simulink model "a"  (R2022a)
settings: Solver=VariableStepAuto  StartTime=0.0  StopTime=0.1  RelTol=1e-3
libraries: commrandsrc3 x1, dspsrcs4 x1
(part 4 of 4)

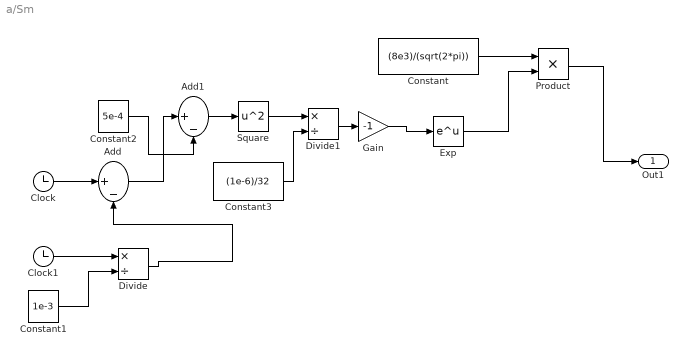
== system a/Sm ==
  Add : Sum  Inputs=|+-
  Add1 : Sum  Inputs=|+-
  Clock : Clock
  Clock1 : Clock
  Constant : Constant  Value=(8e3)/(sqrt(2*pi))
  Constant1 : Constant  Value=1e-3
  Constant2 : Constant  Value=5e-4
  Constant3 : Constant  Value=(1e-6)/32
  Divide : Product  Inputs=*/
  Divide1 : Product  Inputs=*/
  Exp : Math
  Gain : Gain  Gain=-1
  Product : Product
  Square : Math  Operator=square
  Out1 : Outport
  wires:
  Constant/1 -> Product/1
  Exp/1 -> Product/2
  Clock/1 -> Add/1
  Clock1/1 -> Divide/1
  Constant1/1 -> Divide/2
  Divide/1 -> Add/2
  Constant2/1 -> Add1/2
  Add/1 -> Add1/1
  Add1/1 -> Square/1
  Square/1 -> Divide1/1
  Constant3/1 -> Divide1/2
  Divide1/1 -> Gain/1
  Gain/1 -> Exp/1
  Product/1 -> Out1/1

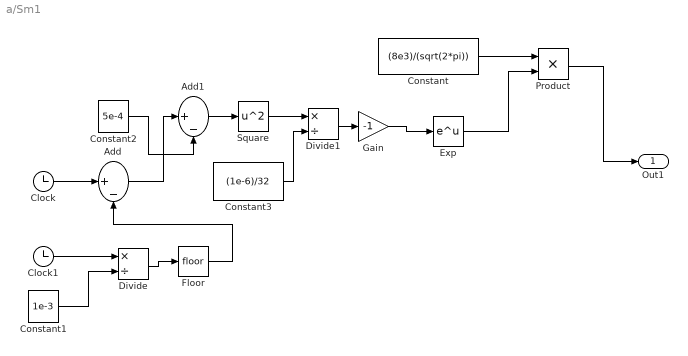
== system a/Sm1 ==
  Add : Sum  Inputs=|+-
  Add1 : Sum  Inputs=|+-
  Clock : Clock
  Clock1 : Clock
  Constant : Constant  Value=(8e3)/(sqrt(2*pi))
  Constant1 : Constant  Value=1e-3
  Constant2 : Constant  Value=5e-4
  Constant3 : Constant  Value=(1e-6)/32
  Divide : Product  Inputs=*/
  Divide1 : Product  Inputs=*/
  Exp : Math
  Floor : Rounding
  Gain : Gain  Gain=-1
  Product : Product
  Square : Math  Operator=square
  Out1 : Outport
  wires:
  Product/1 -> Out1/1
  Gain/1 -> Exp/1
  Divide1/1 -> Gain/1
  Constant3/1 -> Divide1/2
  Square/1 -> Divide1/1
  Add1/1 -> Square/1
  Add/1 -> Add1/1
  Constant2/1 -> Add1/2
  Floor/1 -> Add/2
  Divide/1 -> Floor/1
  Constant1/1 -> Divide/2
  Clock1/1 -> Divide/1
  Clock/1 -> Add/1
  Exp/1 -> Product/2
  Constant/1 -> Product/1
